simulink model "pid_good_result"  (R2021a)
settings: Solver=VariableStepAuto  StartTime=0.0  StopTime=T_s  RelTol=1e-3
values from neighbouring files (symbols this model uses):
  a_x = [0 0 0 0]    [starting_and_end_points.m]
  a_y = [10 40 30 10]    [starting_and_end_points.m]
  a_z = [30 30 30 30]    [starting_and_end_points.m]
  b_x = [0 0 0 0]    [starting_and_end_points.m]
  b_y = [40 30 10 3]    [starting_and_end_points.m]
  b_z = [30 30 30 30]    [starting_and_end_points.m]
  T = 2*max(A)    [starting_and_end_points.m]
libraries: pid_lib x3
settings Model: Creator=Tsehay  LastModifiedBy=Vogayer
settings SolverCC: AlgebraicLoopSolver=TrustRegion
settings DataIOCC: ReturnWorkspaceOutputs=off
settings DebuggingCC: SFMachineParentedDataDiag=warning  ArithmeticOperatorsInVariantConditions=warning
settings SFSimCC: CustomCodeUndefinedFunction=UseInterfaceOnly

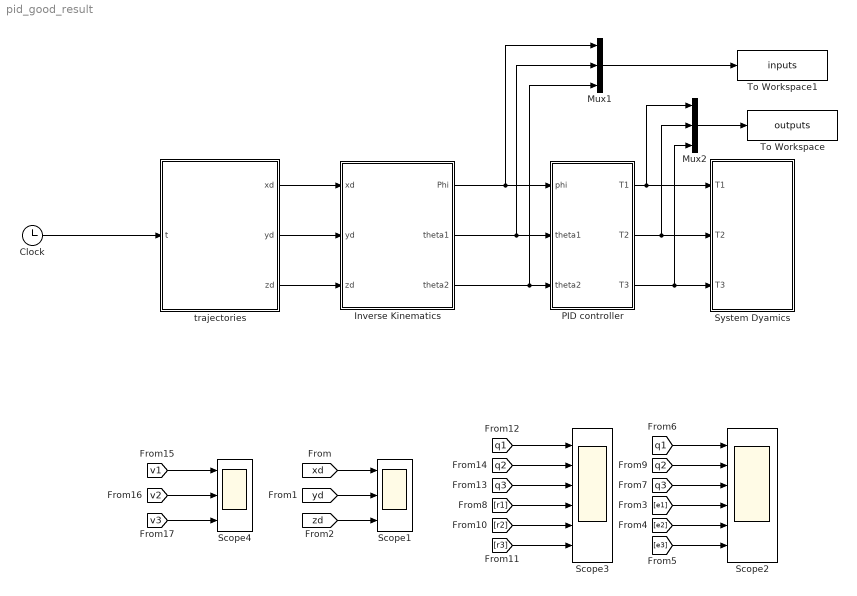
== system pid_good_result ==
  Clock : Clock
  Inverse Kinematics : Subsystem
  Mux1 : Mux  Inputs=3
  Mux2 : Mux  Inputs=3
  PID controller : Subsystem
  Scope1 : Scope  NumInputPorts=3
  Scope2 : Scope  NumInputPorts=6
  Scope3 : Scope  NumInputPorts=6
  Scope4 : Scope  NumInputPorts=3
  System Dyamics : Subsystem
  To Workspace : ToWorkspace  VariableName=outputs  SampleTime=-1
  To Workspace1 : ToWorkspace  VariableName=inputs  SampleTime=-1
  trajectories : Subsystem
  wires:
  [q1] -> Scope2/1
  [q3] -> Scope2/3
  [q2] -> Scope2/2
  [e1] -> Scope2/4
  [e2] -> Scope2/5
  [e3] -> Scope2/6
  [q2] -> Scope3/2
  [r2] -> Scope3/5
  [q1] -> Scope3/1
  [q3] -> Scope3/3
  [r1] -> Scope3/4
  [r3] -> Scope3/6
  [v1] -> Scope4/1
  [v2] -> Scope4/2
  [v3] -> Scope4/3
  Clock/1 -> trajectories/1(t)
  trajectories/1(xd) -> Inverse Kinematics/1(xd)
  trajectories/2(yd) -> Inverse Kinematics/2(yd)
  trajectories/3(zd) -> Inverse Kinematics/3(zd)
  Inverse Kinematics/1(Phi) -> PID controller/1(phi), Mux1/1
  Inverse Kinematics/2(theta1) -> PID controller/2(theta1), Mux1/2
  Inverse Kinematics/3(theta2) -> PID controller/3(theta2), Mux1/3
  PID controller/1(T1) -> Mux2/1, System Dyamics/1(T1)
  PID controller/2(T2) -> Mux2/2, System Dyamics/2(T2)
  PID controller/3(T3) -> Mux2/3, System Dyamics/3(T3)
  [xd] -> Scope1/1
  [yd] -> Scope1/2
  [zd] -> Scope1/3
  Mux2/1 -> To Workspace/1
  Mux1/1 -> To Workspace1/1

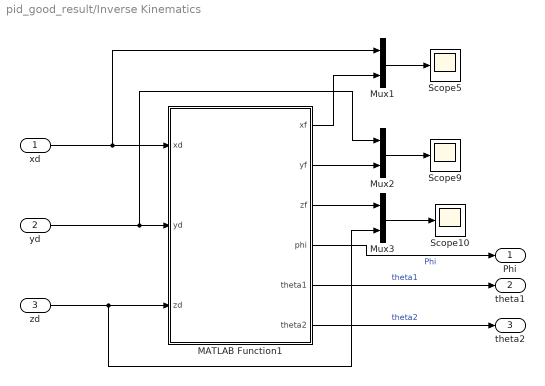
== system pid_good_result/Inverse Kinematics ==
  xd : Inport
  yd : Inport  Port=2
  zd : Inport  Port=3
  MATLAB Function1 : MATLAB Function  TreatAsAtomicUnit=on
  Mux1 : Mux  Inputs=2
  Mux2 : Mux  Inputs=2
  Mux3 : Mux  Inputs=2
  Scope10 : Scope
  Scope5 : Scope
  Scope9 : Scope
  Phi : Outport
  theta1 : Outport  Port=2
  theta2 : Outport  Port=3
  wires:
  yd/1 -> Mux2/1, MATLAB Function1/2(yd)
  xd/1 -> MATLAB Function1/1(xd), Mux1/1
  Mux2/1 -> Scope9/1
  MATLAB Function1/3(zf) -> Mux3/1
  MATLAB Function1/2(yf) -> Mux2/2
  Mux3/1 -> Scope10/1
  Mux1/1 -> Scope5/1
  zd/1 -> Mux3/2, MATLAB Function1/3(zd)
  MATLAB Function1/1(xf) -> Mux1/2
  MATLAB Function1/5(theta1) -> theta1/1  "theta1"
  MATLAB Function1/4(phi) -> Phi/1  "Phi"
  MATLAB Function1/6(theta2) -> theta2/1  "theta2"

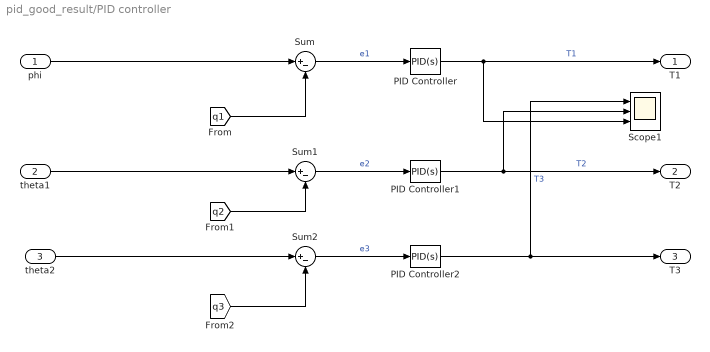
== system pid_good_result/PID controller ==
  phi : Inport
  theta1 : Inport  Port=2
  theta2 : Inport  Port=3
  PID Controller : pid_lib/PID Controller  Controller=PID  Form=Parallel  TimeDomain=Continuous-time  UseExternalTs=off  SampleTime=-1  IntegratorMethod=Forward Euler  FilterMethod=Forward Euler  ControllerParametersSource=internal  P=2.28184982885174  I=1.06824293805434  D=1.19687109159291  UseFilter=on  N=54.5397025421619  TunerSelectOption=Transfer Function Based (PID Tuner App)  InitialConditionSource=internal  InitialConditionForIntegrator=0  InitialConditionForFilter=0  DifferentiatorICPrevScaledInput=0  ExternalReset=none  TrackingMode=off  Kt=1  LimitOutput=off  SatLimitsSource=internal  UpperSaturationLimit=inf  LowerSaturationLimit=-inf  LinearizeAsGain=on  AntiWindupMode=none  Kb=1  POutMin=[]  POutMax=[]  IOutMin=[]  IOutMax=[]  DOutMin=[]  DOutMax=[]  NOutMin=[]  NOutMax=[]  SumOutMin=[]  SumOutMax=[]  SaturationOutMin=[]  SaturationOutMax=[]  PParamMin=[]  PParamMax=[]  IParamMin=[]  IParamMax=[]  DParamMin=[]  DParamMax=[]  NParamMin=[]  NParamMax=[]  KbParamMin=[]  KbParamMax=[]  KtParamMin=[]  KtParamMax=[]  KbOutMin=[]  KbOutMax=[]  KtOutMin=[]  KtOutMax=[]  IntegratorOutMin=[]  IntegratorOutMax=[]  FilterOutMin=[]  FilterOutMax=[]  SumI1OutMin=[]  SumI1OutMax=[]  SumI2OutMin=[]  SumI2OutMax=[]  SumI3OutMin=[]  SumI3OutMax=[]  SumI4OutMin=[]  SumI4OutMax=[]  SumDOutMin=[]  SumDOutMax=[]  DifferentiatorOutMin=[]  DifferentiatorOutMax=[]  FilterDiffOutCoefMin=[]  FilterDiffOutCoefMax=[]  ReciprocalOutMin=[]  ReciprocalOutMax=[]  SumDenOutMin=[]  SumDenOutMax=[]  SumNumOutMin=[]  SumNumOutMax=[]  DivideOutMin=[]  DivideOutMax=[]  UdiffTsProdOutMin=[]  UdiffTsProdOutMax=[]  NTsProdOutMin=[]  NTsProdOutMax=[]  UintegralTsProdOutMin=[]  UintegralTsProdOutMax=[]  UngainTsProdOutMin=[]  UngainTsProdOutMax=[]  IntegratorContinuousStateAttributes=''  IntegratorStateMustResolveToSignalObject=off  IntegratorRTWStateStorageClass=Auto  FilterContinuousStateAttributes=''  FilterStateMustResolveToSignalObject=off  FilterRTWStateStorageClass=Auto  ParallelPVariant=InternalParameters  IdealPVariant=Disabled  IVariant=InternalParameters  DVariant=InternalParameters  IntegratorVariant=Continuous  SatVariant=Disabled  AWVariant=Passthrough  PCopyVariant=Disabled  TRVariant=Disabled  FdbkBlocksVariant=Forward  IdealPFdbkVariant=Disabled  SatFdbkVariant=Disabled  DerivativeFilterVariant=ContFilter  NVariant=InternalParameters  NCopyVariant=Disabled  FilterICVariant=InternalICsFilter  IntegratorICVariant=InternalICs  ExternalResetVariant=Disabled  TRSumVariant=Passthrough  SumFdbkVariant=Disabled  SumVariant=Sum_PID  TsampFilterVariant=InternalTs  TsampNgainVariant=Passthrough  TsampIntegralVariant=Passthrough  ExternalSaturationOutDataTypeStr=Inherit: Same as second input
  PID Controller1 : pid_lib/PID Controller  Controller=PID  Form=Parallel  TimeDomain=Continuous-time  UseExternalTs=off  SampleTime=-1  IntegratorMethod=Forward Euler  FilterMethod=Forward Euler  ControllerParametersSource=internal  P=66.3245976240351  I=108.858021997244  D=7.26461762494016  UseFilter=on  N=389.461376061763  TunerSelectOption=Transfer Function Based (PID Tuner App)  InitialConditionSource=internal  InitialConditionForIntegrator=0  InitialConditionForFilter=0  DifferentiatorICPrevScaledInput=0  ExternalReset=none  TrackingMode=off  Kt=1  LimitOutput=off  SatLimitsSource=internal  UpperSaturationLimit=inf  LowerSaturationLimit=-inf  LinearizeAsGain=on  AntiWindupMode=none  Kb=1  POutMin=[]  POutMax=[]  IOutMin=[]  IOutMax=[]  DOutMin=[]  DOutMax=[]  NOutMin=[]  NOutMax=[]  SumOutMin=[]  SumOutMax=[]  SaturationOutMin=[]  SaturationOutMax=[]  PParamMin=[]  PParamMax=[]  IParamMin=[]  IParamMax=[]  DParamMin=[]  DParamMax=[]  NParamMin=[]  NParamMax=[]  KbParamMin=[]  KbParamMax=[]  KtParamMin=[]  KtParamMax=[]  KbOutMin=[]  KbOutMax=[]  KtOutMin=[]  KtOutMax=[]  IntegratorOutMin=[]  IntegratorOutMax=[]  FilterOutMin=[]  FilterOutMax=[]  SumI1OutMin=[]  SumI1OutMax=[]  SumI2OutMin=[]  SumI2OutMax=[]  SumI3OutMin=[]  SumI3OutMax=[]  SumI4OutMin=[]  SumI4OutMax=[]  SumDOutMin=[]  SumDOutMax=[]  DifferentiatorOutMin=[]  DifferentiatorOutMax=[]  FilterDiffOutCoefMin=[]  FilterDiffOutCoefMax=[]  ReciprocalOutMin=[]  ReciprocalOutMax=[]  SumDenOutMin=[]  SumDenOutMax=[]  SumNumOutMin=[]  SumNumOutMax=[]  DivideOutMin=[]  DivideOutMax=[]  UdiffTsProdOutMin=[]  UdiffTsProdOutMax=[]  NTsProdOutMin=[]  NTsProdOutMax=[]  UintegralTsProdOutMin=[]  UintegralTsProdOutMax=[]  UngainTsProdOutMin=[]  UngainTsProdOutMax=[]  IntegratorContinuousStateAttributes=''  IntegratorStateMustResolveToSignalObject=off  IntegratorRTWStateStorageClass=Auto  FilterContinuousStateAttributes=''  FilterStateMustResolveToSignalObject=off  FilterRTWStateStorageClass=Auto  ParallelPVariant=InternalParameters  IdealPVariant=Disabled  IVariant=InternalParameters  DVariant=InternalParameters  IntegratorVariant=Continuous  SatVariant=Disabled  AWVariant=Passthrough  PCopyVariant=Disabled  TRVariant=Disabled  FdbkBlocksVariant=Forward  IdealPFdbkVariant=Disabled  SatFdbkVariant=Disabled  DerivativeFilterVariant=ContFilter  NVariant=InternalParameters  NCopyVariant=Disabled  FilterICVariant=InternalICsFilter  IntegratorICVariant=InternalICs  ExternalResetVariant=Disabled  TRSumVariant=Passthrough  SumFdbkVariant=Disabled  SumVariant=Sum_PID  TsampFilterVariant=InternalTs  TsampNgainVariant=Passthrough  TsampIntegralVariant=Passthrough  ExternalSaturationOutDataTypeStr=Inherit: Same as second input
  PID Controller2 : pid_lib/PID Controller  Controller=PID  Form=Parallel  TimeDomain=Continuous-time  UseExternalTs=off  SampleTime=-1  IntegratorMethod=Forward Euler  FilterMethod=Forward Euler  ControllerParametersSource=internal  P=92284.2323712411  I=28708337.0909785  D=65.6560213464691  UseFilter=on  N=51610.5658060228  TunerSelectOption=Transfer Function Based (PID Tuner App)  InitialConditionSource=internal  InitialConditionForIntegrator=0  InitialConditionForFilter=0  DifferentiatorICPrevScaledInput=0  ExternalReset=none  TrackingMode=off  Kt=1  LimitOutput=off  SatLimitsSource=internal  UpperSaturationLimit=inf  LowerSaturationLimit=-inf  LinearizeAsGain=on  AntiWindupMode=none  Kb=1  POutMin=[]  POutMax=[]  IOutMin=[]  IOutMax=[]  DOutMin=[]  DOutMax=[]  NOutMin=[]  NOutMax=[]  SumOutMin=[]  SumOutMax=[]  SaturationOutMin=[]  SaturationOutMax=[]  PParamMin=[]  PParamMax=[]  IParamMin=[]  IParamMax=[]  DParamMin=[]  DParamMax=[]  NParamMin=[]  NParamMax=[]  KbParamMin=[]  KbParamMax=[]  KtParamMin=[]  KtParamMax=[]  KbOutMin=[]  KbOutMax=[]  KtOutMin=[]  KtOutMax=[]  IntegratorOutMin=[]  IntegratorOutMax=[]  FilterOutMin=[]  FilterOutMax=[]  SumI1OutMin=[]  SumI1OutMax=[]  SumI2OutMin=[]  SumI2OutMax=[]  SumI3OutMin=[]  SumI3OutMax=[]  SumI4OutMin=[]  SumI4OutMax=[]  SumDOutMin=[]  SumDOutMax=[]  DifferentiatorOutMin=[]  DifferentiatorOutMax=[]  FilterDiffOutCoefMin=[]  FilterDiffOutCoefMax=[]  ReciprocalOutMin=[]  ReciprocalOutMax=[]  SumDenOutMin=[]  SumDenOutMax=[]  SumNumOutMin=[]  SumNumOutMax=[]  DivideOutMin=[]  DivideOutMax=[]  UdiffTsProdOutMin=[]  UdiffTsProdOutMax=[]  NTsProdOutMin=[]  NTsProdOutMax=[]  UintegralTsProdOutMin=[]  UintegralTsProdOutMax=[]  UngainTsProdOutMin=[]  UngainTsProdOutMax=[]  IntegratorContinuousStateAttributes=''  IntegratorStateMustResolveToSignalObject=off  IntegratorRTWStateStorageClass=Auto  FilterContinuousStateAttributes=''  FilterStateMustResolveToSignalObject=off  FilterRTWStateStorageClass=Auto  ParallelPVariant=InternalParameters  IdealPVariant=Disabled  IVariant=InternalParameters  DVariant=InternalParameters  IntegratorVariant=Continuous  SatVariant=Disabled  AWVariant=Passthrough  PCopyVariant=Disabled  TRVariant=Disabled  FdbkBlocksVariant=Forward  IdealPFdbkVariant=Disabled  SatFdbkVariant=Disabled  DerivativeFilterVariant=ContFilter  NVariant=InternalParameters  NCopyVariant=Disabled  FilterICVariant=InternalICsFilter  IntegratorICVariant=InternalICs  ExternalResetVariant=Disabled  TRSumVariant=Passthrough  SumFdbkVariant=Disabled  SumVariant=Sum_PID  TsampFilterVariant=InternalTs  TsampNgainVariant=Passthrough  TsampIntegralVariant=Passthrough  ExternalSaturationOutDataTypeStr=Inherit: Same as second input
  Scope1 : Scope  NumInputPorts=3
  Sum : Sum  Inputs=|+-
  Sum1 : Sum  Inputs=|+-
  Sum2 : Sum  Inputs=|+-
  T1 : Outport
  T2 : Outport  Port=2
  T3 : Outport  Port=3
  wires:
  Sum1/1 -> PID Controller1/1  "e2"
  Sum2/1 -> PID Controller2/1  "e3"
  theta2/1 -> Sum2/1
  [q3] -> Sum2/2
  [q1] -> Sum/2
  Sum/1 -> PID Controller/1  "e1"
  PID Controller2/1 -> Scope1/1, T3/1  "T3"
  phi/1 -> Sum/1
  theta1/1 -> Sum1/1
  PID Controller/1 -> T1/1, Scope1/3  "T1"
  [q2] -> Sum1/2
  PID Controller1/1 -> Scope1/2, T2/1  "T2"

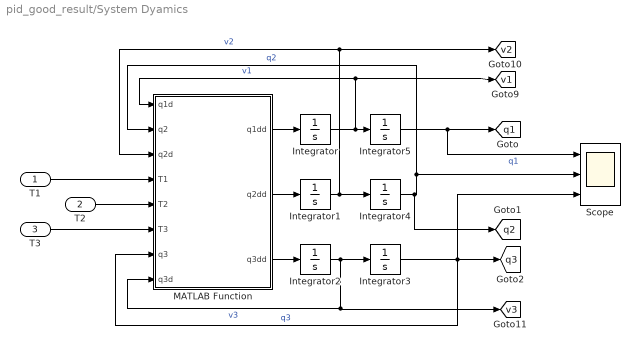
== system pid_good_result/System Dyamics ==
  T1 : Inport
  T2 : Inport  Port=2
  T3 : Inport  Port=3
  Integrator : Integrator
  Integrator1 : Integrator
  Integrator2 : Integrator
  Integrator3 : Integrator  InitialCondition=pi/10
  Integrator4 : Integrator  InitialCondition=pi/6
  Integrator5 : Integrator  InitialCondition=pi/4
  MATLAB Function : MATLAB Function  TreatAsAtomicUnit=on
  Scope : Scope  NumInputPorts=3
  tag scope: q1=global, q2=global, q3=global, v1=global, v2=global, v3=global
  wires:
  Integrator5/1 -> [q1], Scope/1  "q1"
  Integrator4/1 -> Scope/2, MATLAB Function/2(q2), [q2]  "q2"
  MATLAB Function/1(q1dd) -> Integrator/1
  Integrator/1 -> MATLAB Function/1(q1d), [v1], Integrator5/1  "v1"
  Integrator2/1 -> Integrator3/1, [v3], MATLAB Function/8(q3d)  "v3"
  T2/1 -> MATLAB Function/5(T2)
  Integrator3/1 -> MATLAB Function/7(q3), [q3], Scope/3  "q3"
  MATLAB Function/3(q3dd) -> Integrator2/1
  MATLAB Function/2(q2dd) -> Integrator1/1
  Integrator1/1 -> Integrator4/1, [v2], MATLAB Function/3(q2d)  "v2"
  T3/1 -> MATLAB Function/6(T3)
  T1/1 -> MATLAB Function/4(T1)

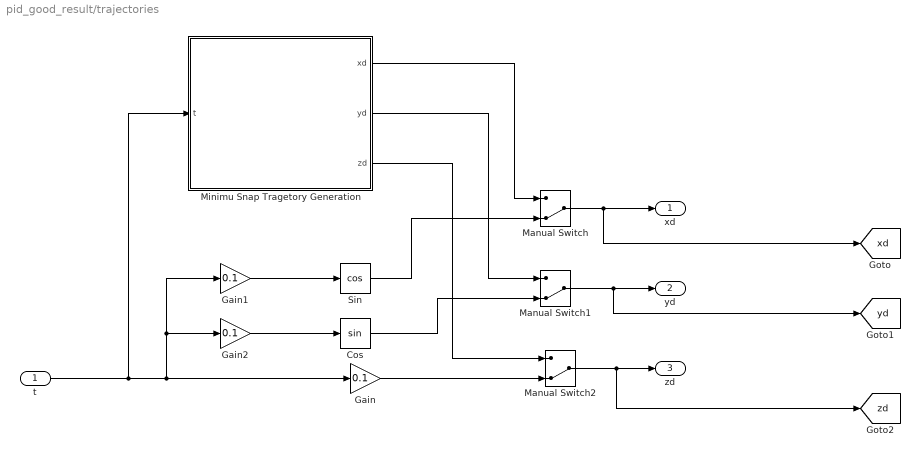
== system pid_good_result/trajectories ==
  t : Inport
  Cos : Trigonometry
  Gain : Gain  Gain=0.1
  Gain1 : Gain  Gain=0.1
  Gain2 : Gain  Gain=0.1
  Manual Switch : ManualSwitch  CurrentSetting=0
  Manual Switch1 : ManualSwitch  CurrentSetting=0
  Manual Switch2 : ManualSwitch  CurrentSetting=0
  Minimu Snap Tragetory Generation : Subsystem
  Sin : Trigonometry  Operator=cos
  xd : Outport
  yd : Outport  Port=2
  zd : Outport  Port=3
  tag scope: xd=global, yd=global, zd=global
  wires:
  Cos/1 -> Manual Switch1/2
  Gain/1 -> Manual Switch2/2
  t/1 -> Minimu Snap Tragetory Generation/1(t), Gain1/1, Gain2/1, Gain/1
  Minimu Snap Tragetory Generation/3(zd) -> Manual Switch2/1
  Minimu Snap Tragetory Generation/1(xd) -> Manual Switch/1
  Minimu Snap Tragetory Generation/2(yd) -> Manual Switch1/1
  Gain1/1 -> Sin/1
  Sin/1 -> Manual Switch/2
  Gain2/1 -> Cos/1
  Manual Switch/1 -> [xd], xd/1
  Manual Switch2/1 -> [zd], zd/1
  Manual Switch1/1 -> [yd], yd/1

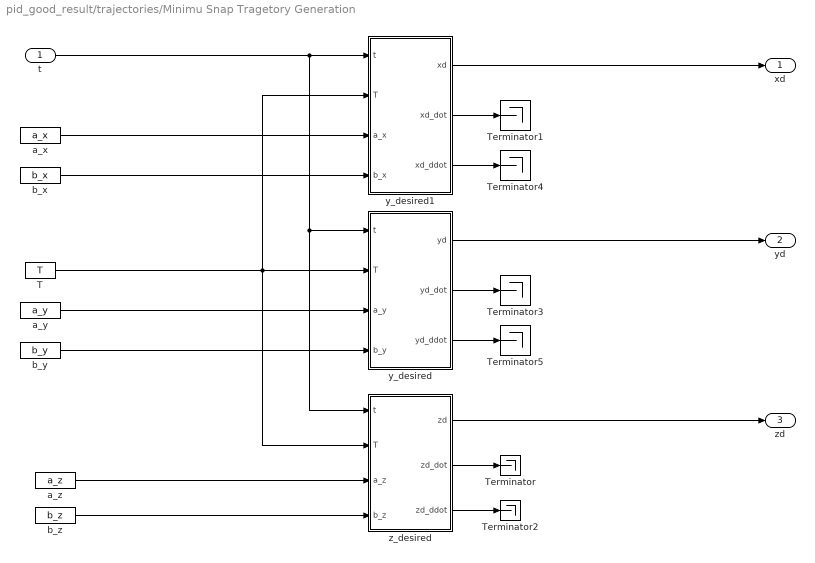
== system pid_good_result/trajectories/Minimu Snap Tragetory Generation ==
  t : Inport
  " z_desired" : MATLAB Function  TreatAsAtomicUnit=on
  T : Constant  Value=T
  Terminator{,1..5} (6 alike) : Terminator
  a_x : Constant  Value=a_x
  a_y : Constant  Value=a_y
  a_z : Constant  Value=a_z
  b_x : Constant  Value=b_x
  b_y : Constant  Value=b_y
  b_z : Constant  Value=b_z
  y_desired : MATLAB Function  TreatAsAtomicUnit=on
  y_desired1 : MATLAB Function  TreatAsAtomicUnit=on
  xd : Outport
  yd : Outport  Port=2
  zd : Outport  Port=3
  wires:
  " z_desired"/3(zd_ddot) -> Terminator2/1
  " z_desired"/2(zd_dot) -> Terminator/1
  t/1 -> y_desired1/1(t), " z_desired"/1(t), y_desired/1(t)
  y_desired/2(yd_dot) -> Terminator3/1
  a_z/1 -> " z_desired"/3(a_z)
  T/1 -> y_desired1/2(T), " z_desired"/2(T), y_desired/2(T)
  y_desired1/1(xd) -> xd/1
  y_desired/1(yd) -> yd/1
  a_y/1 -> y_desired/3(a_y)
  b_z/1 -> " z_desired"/4(b_z)
  y_desired1/2(xd_dot) -> Terminator1/1
  " z_desired"/1(zd) -> zd/1
  b_y/1 -> y_desired/4(b_y)
  y_desired/3(yd_ddot) -> Terminator5/1
  y_desired1/3(xd_ddot) -> Terminator4/1
  a_x/1 -> y_desired1/3(a_x)
  b_x/1 -> y_desired1/4(b_x)

== matlab function pid_good_result/Inverse Kinematics/MATLAB Function1 ==
  data: xd input; xf output; yd input; zd input; yf output; zf output; phi output; theta1 output; theta2 output
function [xf,yf,zf,phi,theta1,theta2] = fcn(xd,yd,zd)
l1=0.25;l2=4;l3=4;
phi=atan2(yd,xd);
r=sqrt(xd^2 + yd^2);
c2 = (r^2 + (zd-l1)^2 - l2^2 - l3^2)/(2*l2*l3);
s2=sqrt(1 - c2^2);
theta2=atan2(s2,c2);
beta=atan((l3*sin(theta2))/(l2 + l3*cos(theta2)));
gama=atan((zd-l1)/r);
theta1=gama-beta;
rf=l2*cos(theta1) + l3*cos((theta1+theta2));
zf=l1+(l2*sin(theta1) + l3*sin(theta1+theta2));
xf=rf*cos(phi);
yf=rf*sin(phi);

== matlab function pid_good_result/System Dyamics/MATLAB Function ==
  data: q1d input; q1dd output; q2 input; q2d input; T1 input; T2 input; T3 input; q3 input; q3d input; q2dd output; q3dd output
function [q1dd, q2dd, q3dd] = fcn(q1d,q2,q2d,T1, T2, T3, q3, q3d)

q1dd=(0.346544E1+0.1E1.*cos(2.*q2)+0.141658E1.*cos(q3)+(-0.154436E0).*cos(2.* ...
  (q2+q3))+0.141658E1.*cos(2.*q2+q3)).^(-1).*(0.457585E2.*T1+cos(q2).*( ...
  0.4E1.*q1d.*q2d.*sin(q2)+0.283317E1.*q1d.*q3d.*sin(q2+q3))+q1d.*(( ...
  -0.308873E0).*q2d+(-0.308873E0).*q3d).*sin(2.*(q2+q3))+0.283317E1.*q1d.* ...
  q2d.*sin(2.*q2+q3));

q2dd=((-0.358251E1)+0.1E1.*cos(q3).^2).^(-1).*((-0.49302E2).*T2+0.49302E2.* ...
  T3+0.144803E-13.*cos(q2+q3)+(-0.152628E1).*q2d.^2.*sin(q3)+(-0.305257E1) ...
  .*q2d.*q3d.*sin(q3)+cos(q2).*(0.119691E3+0.215488E1.*q1d.^2.*sin(q2)+ ...
  q1d.^2.*((-0.152628E1)+(-1.E0).*cos(q3)).*sin(q2+q3))+cos(q3).*( ...
  0.32302E2.*T3+(-0.351613E2).*cos(q2+q3)+(-1.E0).*q2d.^2.*sin(q3)+ ...
  0.10902E0.*q1d.^2.*sin(2.*(q2+q3)))+0.152628E1.*q1d.^2.*sin(2.*q2+q3));

q3dd=(0.343344E-2+(-0.958388E-3).*cos(q3).^2).^(-1).*(0.619157E-1.*( ...
  0.193675E1+0.1E1.*cos(q3)).*(T3+(-0.108852E1).*cos(q2+q3)+(-0.309578E-1) ...
  .*q2d.^2.*sin(q3)+(-0.309578E-1).*q1d.^2.*cos(q2).*sin(q2+q3)+ ...
  0.337503E-2.*q1d.^2.*sin(2.*(q2+q3)))+(-0.309578E-1).*(0.152628E1+0.1E1.* ...
  cos(q3)).*(T2+(-0.108852E1).*cos(q2+q3)+cos(q2).*((-0.242771E1)+( ...
  -0.437077E-1).*q1d.^2.*sin(q2))+0.619157E-1.*q2d.*q3d.*sin(q3)+ ...
  0.337503E-2.*q1d.^2.*sin(2.*(q2+q3))+(-0.309578E-1).*q1d.^2.*sin(2.*q2+q3) ...
  ));

== matlab function pid_good_result/trajectories/Minimu Snap Tragetory Generation/y_desired1 ==
  data: t input; T input; xd output; xd_dot output; xd_ddot output; a_x input; b_x input
function [xd,xd_dot,xd_ddot] = fcn(t,T,a_x,b_x)
if(t<=T(1,1))
T0=0;Tf=T(1,1);
a=a_x(1,1); b=b_x(1,1);
elseif(t>T(1,1)&& t<=T(2,1)+T(1,1))
T0=T(1,1);Tf=T(2,1)+T(1,1);
a=a_x(2,1); b=b_x(2,1);
elseif (t>T(2,1)+T(1,1)&& t<=T(3,1) + T(2,1)+T(1,1))
T0=T(2,1)+T(1,1);Tf=T(3,1)+ T(2,1)+T(1,1);
a=a_x(3,1); b=b_x(3,1);
else
T0=T(3,1)+ T(2,1)+T(1,1);Tf=T(4,1) + T(3,1)+ T(2,1)+T(1,1);
a=a_x(4,1); b=b_x(4,1);
end
B=[a;b;0;0;0;0;0;0];
A=[T0^6     T0^5     T0^4     T0^3    T0^2  T0^1  1;
   Tf^6     Tf^5     Tf^4     Tf^3    Tf^2  Tf^1  1;
   6*T0^5   5*T0^4   4*T0^3   3*T0^2  2*T0  1     0;
   6*Tf^5   5*Tf^4   4*Tf^3   3*Tf^2  2*Tf  1     0;
   30*T0^4  20*T0^3  12*T0^2  6*T0    2     0     0;
   30*Tf^4  20*Tf^3  12*Tf^2  6*Tf    2     0     0;
   120*T0^3  60*T0^2  24*T0   6       2     0     0;
   120*Tf^3  60*Tf^2  24*Tf   6       2     0     0];
C=A\B;
xd=C(1,1)*t^6 + C(2,1)*t^5 + C(3,1)*t^4 + C(4,1)*t^3 + C(5,1)*t^2 + C(6,1)*t + C(7,1);
xd_dot=6*C(1,1)*t^5 + 5*C(2,1)*t^4  + 4*C(3,1)*t^3 + 3*C(4,1)*t^2 + 2*C(5,1)*t + C(6,1);
xd_ddot=30*C(1,1)*t^4 + 20*C(2,1)*t^3  + 12*C(3,1)*t^2 + 6*C(4,1)*t + 2*C(5,1);

== matlab function pid_good_result/trajectories/Minimu Snap Tragetory Generation/y_desired ==
  data: t input; T input; yd output; yd_dot output; yd_ddot output; a_y input; b_y input
function [yd,yd_dot,yd_ddot] = fcn(t,T,a_y,b_y)
if(t<=T(1,1))
T0=0;Tf=T(1,1);
a=a_y(1,1); b=b_y(1,1);
elseif(t>T(1,1)&& t<=T(2,1)+T(1,1))
T0=T(1,1);Tf=T(2,1)+T(1,1);
a=a_y(2,1); b=b_y(2,1);
elseif (t>T(2,1)+T(1,1)&& t<=T(3,1) + T(2,1)+T(1,1))
T0=T(2,1)+T(1,1);Tf=T(3,1)+ T(2,1)+T(1,1);
a=a_y(3,1); b=b_y(3,1);
else
T0=T(3,1)+ T(2,1)+T(1,1);Tf=T(4,1) + T(3,1)+ T(2,1)+T(1,1);
a=a_y(4,1); b=b_y(4,1);
end
B=[a;b;0;0;0;0;0;0];
A=[T0^6     T0^5     T0^4     T0^3    T0^2  T0^1  1;
   Tf^6     Tf^5     Tf^4     Tf^3    Tf^2  Tf^1  1;
   6*T0^5   5*T0^4   4*T0^3   3*T0^2  2*T0  1     0;
   6*Tf^5   5*Tf^4   4*Tf^3   3*Tf^2  2*Tf  1     0;
   30*T0^4  20*T0^3  12*T0^2  6*T0    2     0     0;
   30*Tf^4  20*Tf^3  12*Tf^2  6*Tf    2     0     0;
   120*T0^3  60*T0^2  24*T0   6       2     0     0;
   120*Tf^3  60*Tf^2  24*Tf   6       2     0     0];
C=A\B;
yd=C(1,1)*t^6 + C(2,1)*t^5 + C(3,1)*t^4 + C(4,1)*t^3 + C(5,1)*t^2 + C(6,1)*t + C(7,1);
yd_dot=6*C(1,1)*t^5 + 5*C(2,1)*t^4  + 4*C(3,1)*t^3 + 3*C(4,1)*t^2 + 2*C(5,1)*t + C(6,1);
yd_ddot=30*C(1,1)*t^4 + 20*C(2,1)*t^3  + 12*C(3,1)*t^2 + 6*C(4,1)*t + 2*C(5,1);

== matlab function pid_good_result/trajectories/Minimu Snap Tragetory Generation/ z_desired ==
  data: t input; T input; zd output; zd_dot output; zd_ddot output; a_z input; b_z input
function [zd,zd_dot,zd_ddot] = fcn(t,T,a_z,b_z)
if(t<=T(1,1))
T0=0;Tf=T(1,1);
a=a_z(1,1); b=b_z(1,1);
elseif(t>T(1,1)&& t<=T(2,1)+T(1,1))
T0=T(1,1);Tf=T(2,1)+T(1,1);
a=a_z(2,1); b=b_z(2,1);
elseif (t>T(2,1)+T(1,1)&& t<=T(3,1) + T(2,1)+T(1,1))
T0=T(2,1)+T(1,1);Tf=T(3,1)+ T(2,1)+T(1,1);
a=a_z(3,1); b=b_z(3,1);
else
T0=T(3,1)+ T(2,1)+T(1,1);Tf=T(4,1) + T(3,1)+ T(2,1)+T(1,1);
a=a_z(4,1); b=b_z(4,1);
end
B=[a;b;0;0;0;0;0;0];
A=[T0^6     T0^5     T0^4     T0^3    T0^2  T0^1  1;
   Tf^6     Tf^5     Tf^4     Tf^3    Tf^2  Tf^1  1;
   6*T0^5   5*T0^4   4*T0^3   3*T0^2  2*T0  1     0;
   6*Tf^5   5*Tf^4   4*Tf^3   3*Tf^2  2*Tf  1     0;
   30*T0^4  20*T0^3  12*T0^2  6*T0    2     0     0;
   30*Tf^4  20*Tf^3  12*Tf^2  6*Tf    2     0     0;
   120*T0^3  60*T0^2  24*T0   6       2     0     0;
   120*Tf^3  60*Tf^2  24*Tf   6       2     0     0];
C=A\B;
zd=C(1,1)*t^6 + C(2,1)*t^5 + C(3,1)*t^4 + C(4,1)*t^3 + C(5,1)*t^2 + C(6,1)*t + C(7,1);
zd_dot=6*C(1,1)*t^5 + 5*C(2,1)*t^4  + 4*C(3,1)*t^3 + 3*C(4,1)*t^2 + 2*C(5,1)*t + C(6,1);
zd_ddot=30*C(1,1)*t^4 + 20*C(2,1)*t^3  + 12*C(3,1)*t^2 + 6*C(4,1)*t + 2*C(5,1);
